simulink model "Concatenate7"  (R2017b)
settings: Solver=FixedStepAuto  StartTime=0.0  StopTime=0  FixedStep=0.1  MaxStep=1  RelTol=1e-3  EnableMultiTasking=on
settings Model: Creator=arnaud  LastModifiedBy=ktrinh
settings DataIOCC: LimitDataPoints=on  SaveFormat=Structure
settings OptimizationCC: LifeSpan=inf
settings DebuggingCC: SolverPrmCheckMsg=warning  SFUnexpectedBacktrackingDiag=warning  SFNoUnconditionalDefaultTransitionDiag=warning  SFExecutionAtInitializationDiag=none
settings HardwareCC: ProdBitPerPointer=32  ProdBitPerSizeT=32  ProdBitPerPtrDiffT=32  ProdLargestAtomicFloat=None  ProdIntDivRoundTo=Undefined  ProdEndianess=Unspecified  ProdWordSize=32  ProdHWDeviceType=32-bit Generic
settings ModelReferenceCC: PropagateSignalLabelsOutOfModel=off
settings CodeAppCC: StateflowObjectComments=on
settings GRTTargetCC: TargetLangStandard=C89/C90 (ANSI)  GeneratePreprocessorConditionals=Disable all
settings ConfigComp: CovMetricSettings=dw  CovHtmlReporting=on  CovSaveCumulativeToWorkspaceVar=on  CovSaveSingleToWorkspaceVar=on  CovExternalEMLEnable=off  CovSFcnEnable=off

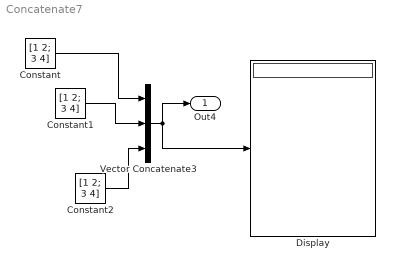
== system Concatenate7 ==
  Constant : Constant  Value=[1 2; 3 4]
  Constant1 : Constant  Value=[1 2; 3 4]
  Constant2 : Constant  Value=[1 2; 3 4]
  Display : Display
  Vector Concatenate3 : Concatenate  NumInputs=3  Mode=Multidimensional array
  Out4 : Outport
  wires:
  Vector Concatenate3/1 -> Out4/1, Display/1
  Constant/1 -> Vector Concatenate3/1
  Constant1/1 -> Vector Concatenate3/2
  Constant2/1 -> Vector Concatenate3/3
